simulink model "Test_TransmSfunc"  (R2018b)
settings: Solver=ode3  StartTime=0.0  StopTime=1  FixedStep=0.001  RelTol=1e-3
PreLoadFcn:
  | Transm_Ptbs_V1_BusInfo
settings Model: Creator=E00026  LastModifiedBy=E00026
settings DataIOCC: SaveFormat=Array  SaveOutput=off  SaveTime=off

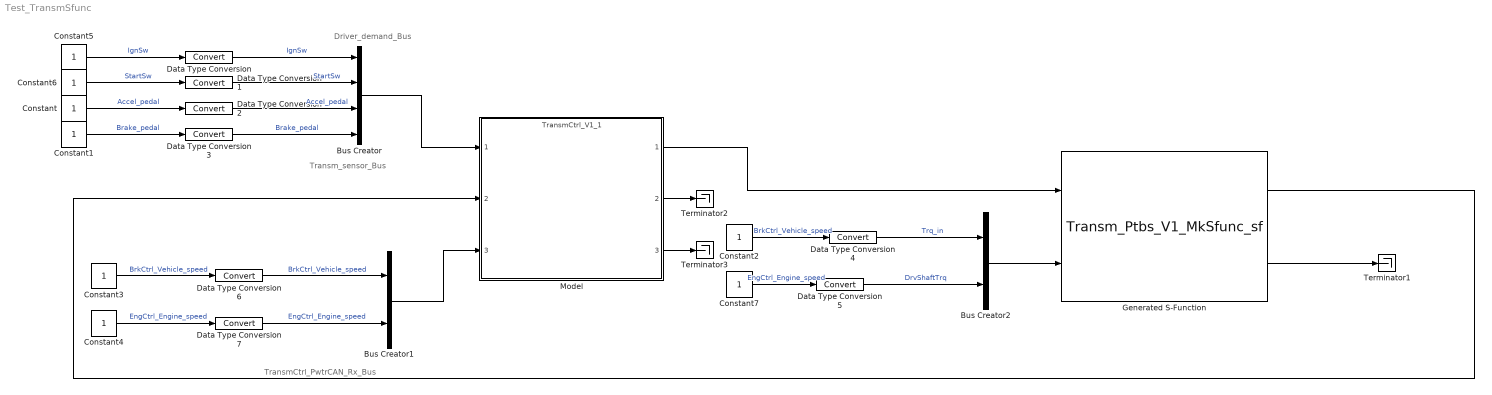
== system Test_TransmSfunc ==
  note: Transm_sensor_Bus
  note: Driver_demand_Bus
  note: TransmCtrl_PwtrCAN_Rx_Bus
  Bus Creator : BusCreator  Inputs=4  OutDataTypeStr=Bus: Driver_demand_Bus
  Bus Creator1 : BusCreator  Inputs=2  OutDataTypeStr=Bus: TransmCtrl_PwtrCAN_Rx_Bus
  Bus Creator2 : BusCreator  Inputs=2  OutDataTypeStr=Bus: Transm_in_Bus
  Constant{,1..7} (8 alike) : Constant
  Data Type Conversion{,1..7} (8 alike) : DataTypeConversion
  Generated S-Function : S-Function  FunctionName=Transm_Ptbs_V1_MkSfunc_sf  Parameters=sfcnParam1, sfcnParam2, sfcnParam3, sfcnParam4, sfcnParam5, sfcnParam6, sfcnParam7, sfcnParam8, sfcnParam9, sfcnParam10, sfcnParam11, sfcnParam12, sfcnParam13, sfcnParam14, sfcnParam15, sfcnParam16, sfcnParam17, sfcnParam18  SFunctionModules=""  SFunctionDeploymentMode=off  EnableBusSupport=off  mask{rtw_sf_name=Transm_Ptbs_V1_MkSfunc_sf, showVar=off, sfcnParam1=[-1.0, 0.0, 1.0, 2.0, 3.0, 4.0, 5.0], sfcnParam2=[0.0], sfcnParam3=[0.3], sfcnParam4=[0.128, 0.01, 0.128, 0.1, 0.062, 0.028, 0.01], sfcnParam5=[5000.0], sfcnParam6=[-4.47, 1.0, 4.47, 2.47, 1.47, 1.0, 0.8], sfcnParam7=[0.2], sfcnParam8=[0.03], sfcnParam9=[0.003, 0.001, 0.003, 0.0025, 0.002, 0.001, 0.001], sfcnParam10=[1.0], sfcnParam11=[0.9, 0.9, 0.9, 0.9, 0.9, 0.95, 0.95], sfcnParam12=[0.4], sfcnParam13=[0.6], sfcnParam14=[0.0], sfcnParam15=[0.0], sfcnParam16=[0.02], sfcnParam17=[1.0E-6], sfcnParam18=[0.15]}
      mask prompts: rtw_sf_name "Simulink:masks:GenSFuncName_MP"; showVar "Simulink:masks:GenSFuncShowModuleList_MP"; sfcnParam1 "AutomatedManualTransmission_G:"; sfcnParam2 "AutomatedManualTransmission_G_o:"; sfcnParam3 "AutomatedManualTransmission_Jin:"; sfcnParam4 "AutomatedManualTransmission_Jout:"; sfcnParam5 "AutomatedManualTransmission_K_c:"; sfcnParam6 "AutomatedManualTransmission_N:"; sfcnParam7 "AutomatedManualTransmission_R:"; sfcnParam8 "AutomatedManualTransmission_bin:"; sfcnParam9 "AutomatedManualTransmission_bout:"; sfcnParam10 "CompareToConstant_const:"; sfcnParam11 "AutomatedManualTransmission_eta:"; sfcnParam12 "AutomatedManualTransmission_muk:"; sfcnParam13 "AutomatedManualTransmission_mus:"; sfcnParam14 "AutomatedManualTransmission_omegain_o:"; sfcnParam15 "AutomatedManualTransmission_omegaout_o:"; sfcnParam16 "AutomatedManualTransmission_tauc:"; sfcnParam17 "div0protectabspoly1_thresh:"; sfcnParam18 "AutomatedManualTransmission_ts:"
      mask help: Simulink:masks:GenSFuncDesc_MD
      mask init:
      | displist = '';
      | if ~strcmp(get_param(gcb, 'FunctionName'), rtw_sf_name);
      |   set_param(gcb, 'FunctionName', rtw_sf_name);
      | end
      | % Check if we are generating code
      | rtw_mode = false;
      | if strcmpi(get_param(bdroot(gcb),'SimulationStatus'),'Initializing')
      | 	rtw_mode = strcmpi(get_param(bdroot(gcb),'BuildingRTWCode'),'on') && ...
      | 		~strcmpi(get_param(bdroot(gcb),'TargetStyle'),'SimulationTarget');
      | end
      | if showVar || rtw_mode
      | 	if exist('rtwsfunc') == 2 | exist('rtwsfunc') == 6
      | 		tmplist = rtwsfunc(rtw_sf_name,gcb);
      | 		tmplist = DAStudio.message('Simulink:masks:GenSFuncListOfModules_IC', tmplist);
      | 	elseif showVar
      | 		tmplist1 = DAStudio.message('Simulink:masks:GenSFuncListOfModules_IC', '');
      |         tmplist2 = DAStudio.message('Simulink:masks:GenSFuncNotLicensed_IC');
      |         tmplist = [tmplist1 tmplist2];
      |  	end
      | end
      | if showVar
      |   displist = tmplist;
      | end
      settings: CopyFcn=|
      | if ~strcmp(get_param(gcb,'Linkstatus'),'none') && ...
      | ~strcmp(get_param(gcb,'Linkstatus'),'implicit')
      |   set_param(gcb,'LinkStatus','none');
      | end
      mask Help: eval('feval(''rtwprivate'',''rtwhelpview'',''rtw_sfcn_block'')');
      mask Display:
      | port_label('input',1,'TransmCtrl');
      | port_label('input',2,'Transm_in');
      | port_label('output',1,'Transm_sensor');
      | port_label('output',2,'Transm_out');
  Model : ModelReference  ModelNameDialog=TransmCtrl_V1_1.slx  SimulationMode=Normal  ModelReferenceVersion=1.0.43
  Terminator1 : Terminator
  Terminator2 : Terminator
  Terminator3 : Terminator
  wires:
  Generated S-Function/1 -> Model/2
  Model/1 -> Generated S-Function/1
  Bus Creator/1 -> Model/1
  Data Type Conversion1/1 -> Bus Creator/2  "StartSw"
  Constant5/1 -> Data Type Conversion/1  "IgnSw"
  Constant6/1 -> Data Type Conversion1/1  "StartSw"
  Data Type Conversion/1 -> Bus Creator/1  "IgnSw"
  Constant1/1 -> Data Type Conversion3/1  "Brake_pedal"
  Data Type Conversion2/1 -> Bus Creator/3  "Accel_pedal"
  Data Type Conversion3/1 -> Bus Creator/4  "Brake_pedal"
  Constant/1 -> Data Type Conversion2/1  "Accel_pedal"
  Data Type Conversion6/1 -> Bus Creator1/1  "BrkCtrl_Vehicle_speed"
  Data Type Conversion7/1 -> Bus Creator1/2  "EngCtrl_Engine_speed"
  Constant3/1 -> Data Type Conversion6/1  "BrkCtrl_Vehicle_speed"
  Constant4/1 -> Data Type Conversion7/1  "EngCtrl_Engine_speed"
  Bus Creator1/1 -> Model/3
  Generated S-Function/2 -> Terminator1/1
  Model/2 -> Terminator2/1
  Model/3 -> Terminator3/1
  Constant7/1 -> Data Type Conversion5/1  "EngCtrl_Engine_speed"
  Constant2/1 -> Data Type Conversion4/1  "BrkCtrl_Vehicle_speed"
  Data Type Conversion5/1 -> Bus Creator2/2  "DrvShaftTrq"
  Data Type Conversion4/1 -> Bus Creator2/1  "Trq_in"
  Bus Creator2/1 -> Generated S-Function/2
